simulink model "modelo"  (R2020a)
settings: Solver=FixedStepAuto  StartTime=0.0  StopTime=0.05  FixedStep=100e-9  RelTol=1e-3
values from neighbouring files (symbols this model uses):
  c1 = 220e-6    (= 0.00022)    [Untitled.m]
  c2 = 220e-6    (= 0.00022)    [Untitled.m]
  lb = 33e-6    (= 3.3e-05)    [Untitled.m]
  lr = 1.7e-6    (= 1.7e-06)    [Untitled.m]
  rb = 0.010    (= 0.01)    [Untitled.m]
  sc1 = 0.350    (= 0.35)    [Untitled.m]
  sc2 = 0.350    (= 0.35)    [Untitled.m]
  vb = 3.3    [Untitled.m]
  w = 2*pi*20e3    (= 125663.706144)    [Untitled.m]
libraries: powerlib x27
settings Model: Creator=nunin  LastModifiedBy=nunin

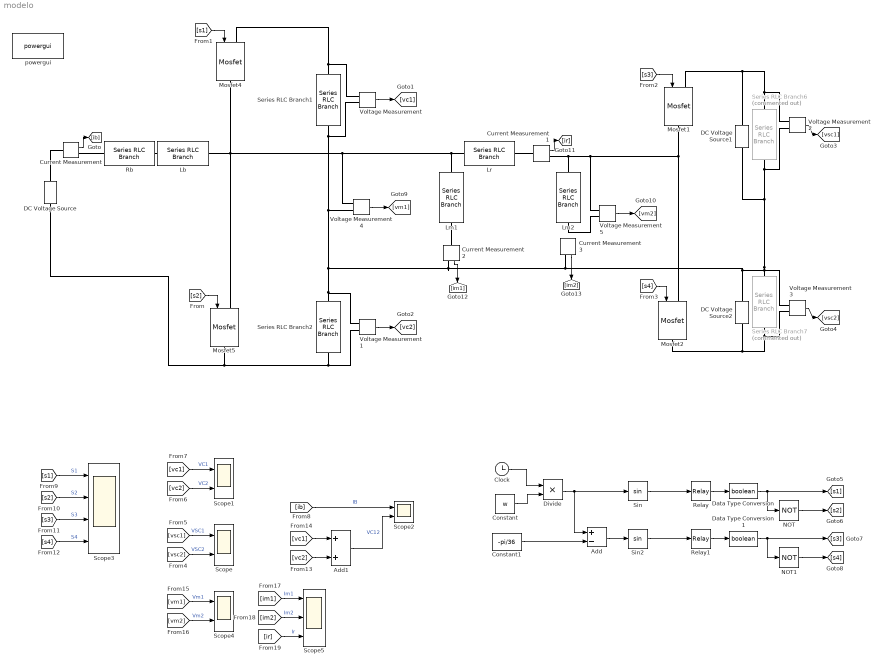
== system modelo ==
  Add : Sum  Inputs=+-
  Add1 : Sum
  Clock : Clock
  Constant : Constant  Value=w
  Constant1 : Constant  Value=-pi/36  VectorParams1D=off
  Current Measurement{,1..3} (4 alike) : powerlib/Measurements/Current Measurement  PhasorSimulation=off  OutputType=Complex  PSBequivalent=0
  DC Voltage Source : powerlib/Electrical Sources/DC Voltage Source  Amplitude=vb  Measurements=None
  DC Voltage Source1 : powerlib/Electrical Sources/DC Voltage Source  Amplitude=vb  Measurements=None
  DC Voltage Source2 : powerlib/Electrical Sources/DC Voltage Source  Amplitude=vb  Measurements=None
  Data Type Conversion : DataTypeConversion  OutDataTypeStr=boolean
  Data Type Conversion1 : DataTypeConversion  OutDataTypeStr=boolean
  Divide : Product  Inputs=**
  Lb : powerlib/Elements/Series RLC Branch  LConnTagsString=__new0  RConnTagsString=__new0  BranchType=L  Resistance=rb  Inductance=lb  SetiL0=off  InitialCurrent=0  Capacitance=1e-6  Setx0=off  InitialVoltage=0  Measurements=None
  Lm1 : powerlib/Elements/Series RLC Branch  LConnTagsString=__new0  RConnTagsString=__new0  BranchType=L  Resistance=rb  Inductance=1  SetiL0=off  InitialCurrent=0  Capacitance=1e-6  Setx0=off  InitialVoltage=0  Measurements=None
  Lm2 : powerlib/Elements/Series RLC Branch  LConnTagsString=__new0  RConnTagsString=__new0  BranchType=L  Resistance=rb  Inductance=1  SetiL0=off  InitialCurrent=0  Capacitance=1e-6  Setx0=off  InitialVoltage=0  Measurements=None
  Lr : powerlib/Elements/Series RLC Branch  LConnTagsString=__new0  RConnTagsString=__new0  BranchType=L  Resistance=rb  Inductance=lr  SetiL0=off  InitialCurrent=0  Capacitance=1e-6  Setx0=off  InitialVoltage=0  Measurements=None
  Mosfet{1..2,4..5} (4 alike) : powerlib/Power Electronics/Mosfet  Ron=1e-9  Lon=0  Rd=1e-9  Vfd=0  IC=0  Rs=1e10  Cs=inf  Measurements=off
  NOT : Logic  Operator=NOT  IconShape=distinctive  AllPortsSameDT=off  OutDataTypeStr=boolean
  NOT1 : Logic  Operator=NOT  IconShape=distinctive  AllPortsSameDT=off  OutDataTypeStr=boolean
  Rb : powerlib/Elements/Series RLC Branch  LConnTagsString=__new0  RConnTagsString=__new0  BranchType=R  Resistance=rb  Inductance=lb  SetiL0=off  InitialCurrent=0  Capacitance=1e-6  Setx0=off  InitialVoltage=0  Measurements=None
  Relay : Relay
  Relay1 : Relay
  Scope{,1..2,4} (4 alike) : Scope  NumInputPorts=2
  Scope3 : Scope  NumInputPorts=4
  Scope5 : Scope  NumInputPorts=3
  Series RLC Branch1 : powerlib/Elements/Series RLC Branch  LConnTagsString=__new0  RConnTagsString=__new0  BranchType=C  Resistance=rb  Inductance=lb  SetiL0=off  InitialCurrent=0  Capacitance=c1  Setx0=on  InitialVoltage=3.3  Measurements=None
  Series RLC Branch2 : powerlib/Elements/Series RLC Branch  LConnTagsString=__new0  RConnTagsString=__new0  BranchType=C  Resistance=rb  Inductance=lb  SetiL0=off  InitialCurrent=0  Capacitance=c2  Setx0=on  InitialVoltage=3.3  Measurements=None
  Series RLC Branch6 : powerlib/Elements/Series RLC Branch  Commented=on  LConnTagsString=__new0  RConnTagsString=__new0  BranchType=C  Resistance=rb  Inductance=lb  SetiL0=off  InitialCurrent=0  Capacitance=sc1  Setx0=on  InitialVoltage=3.3  Measurements=None
  Series RLC Branch7 : powerlib/Elements/Series RLC Branch  Commented=on  LConnTagsString=__new0  RConnTagsString=__new0  BranchType=C  Resistance=rb  Inductance=lb  SetiL0=off  InitialCurrent=0  Capacitance=sc2  Setx0=on  InitialVoltage=3.3  Measurements=None
  Sin : Trigonometry
  Sin2 : Trigonometry
  Voltage Measurement{,1..5} (6 alike) : powerlib/Measurements/Voltage Measurement  PhasorSimulation=off  OutputType=Complex  PSBequivalent=0
  powergui : powerlib/powergui  Priority=1  SimulationMode=Discrete  SampleTime=100e-9  frequency=60  Iterations=50  frequencyindice=0  Pbase=100e6  ErrMax=1e-4  UnitsV=kV  UnitsW=MW  buscounter=0  FunctionMessages=off  echomessages=off  EnableUseOfTLC=off  CurrentSourceSwitches=off  DisableSnubberDevices=off  DisableRonSwitches=off  DisableVfSwitches=off  DisplayEquations=off  AutomaticDiscreteSolvers=off  SolverType=Tustin/Backward Euler (TBE)  Interpol=off  ExternalGateDelay=off  methode=off  Ts=100  x0status=blocks  SPID=on  SwTol=0  HookPort=off  NonlinearTolerance=1e-4  nMaxIteration=100  ContinueOnMaxIteration=off  RestoreLinks=warning  ResistiveCurrentMeasurement=off  Frange=[0:2:500]  Ylog=off  Xlog=on  ShowGrid=off  save=off  variable=ZData  structure=0  ZoomFFT=off  StartTime=0.0  cycles=1  DisplayStyle=1  fundamental=60  FreqAxis=off  MaxFrequency=1000  frequencyindicesteady=1  RmsSteady=1  display=off
  wires:
  Current Measurement/1 -> [ib]
  Voltage Measurement/1 -> [vc1]
  Voltage Measurement1/1 -> [vc2]
  Voltage Measurement2/1 -> [vsc1]
  Voltage Measurement3/1 -> [vsc2]
  Clock/1 -> Divide/1
  Constant/1 -> Divide/2
  Divide/1 -> Add/1, Sin/1
  Constant1/1 -> Add/2
  Add/1 -> Sin2/1
  Sin/1 -> Relay/1
  Sin2/1 -> Relay1/1
  Relay/1 -> Data Type Conversion/1
  Data Type Conversion/1 -> NOT/1, [s1]
  NOT/1 -> [s2]
  NOT1/1 -> [s4]
  Data Type Conversion1/1 -> [s3], NOT1/1
  Relay1/1 -> Data Type Conversion1/1
  [s2] -> Mosfet5/1
  [s4] -> Mosfet2/1
  [s3] -> Mosfet1/1
  [s1] -> Mosfet4/1
  [vsc2] -> Scope/2  "VSC2"
  [vsc1] -> Scope/1  "VSC1"
  [vc2] -> Scope1/2  "VC2"
  [vc1] -> Scope1/1  "VC1"
  [ib] -> Scope2/1  "IB"
  [s1] -> Scope3/1  "S1"
  [s2] -> Scope3/2  "S2"
  [s4] -> Scope3/4  "S4"
  [s3] -> Scope3/3  "S3"
  [vc2] -> Add1/2
  [vc1] -> Add1/1
  Add1/1 -> Scope2/2  "VC12"
  Voltage Measurement4/1 -> [vm1]
  Voltage Measurement5/1 -> [vm2]
  [vm2] -> Scope4/2  "Vm2"
  [vm1] -> Scope4/1  "Vm1"
  Current Measurement1/1 -> [ir]
  Current Measurement2/1 -> [im1]
  Current Measurement3/1 -> [im2]
  [im1] -> Scope5/1  "Im1"
  [im2] -> Scope5/2  "Im2"
  [ir] -> Scope5/3  "Ir"
  connections:
  Rb/LConn1 -- Current Measurement/RConn1
  Current Measurement/LConn1 -- DC Voltage Source/RConn1
  Series RLC Branch1/LConn1 -- Mosfet4/LConn1 -- Voltage Measurement/LConn1
  Series RLC Branch2/RConn1 -- Mosfet5/RConn1 -- DC Voltage Source/LConn1 -- Voltage Measurement1/LConn2
  Lr/LConn1 -- Voltage Measurement4/LConn1 -- Mosfet5/LConn1 -- Mosfet4/RConn1 -- Lb/RConn1 -- Lm1/LConn1
  Voltage Measurement2/LConn1 -- Mosfet1/LConn1 -- DC Voltage Source1/RConn1 -- Series RLC Branch6/LConn1
  Voltage Measurement3/LConn2 -- Mosfet2/RConn1 -- DC Voltage Source2/LConn1 -- Series RLC Branch7/RConn1
  Series RLC Branch2/LConn1 -- Voltage Measurement1/LConn1 -- Current Measurement2/RConn1 -- Current Measurement3/RConn1 -- DC Voltage Source2/RConn1 -- Series RLC Branch7/LConn1 -- DC Voltage Source1/LConn1 -- Voltage Measurement2/LConn2 -- Series RLC Branch6/RConn1 -- Voltage Measurement3/LConn1 -- Voltage Measurement/LConn2 -- Series RLC Branch1/RConn1 -- Voltage Measurement4/LConn2
  Lb/LConn1 -- Rb/RConn1
  Voltage Measurement5/LConn1 -- Mosfet2/LConn1 -- Mosfet1/RConn1 -- Lm2/LConn1 -- Current Measurement1/RConn1
  Current Measurement1/LConn1 -- Lr/RConn1
  Current Measurement2/LConn1 -- Lm1/RConn1
  Lm2/RConn1 -- Voltage Measurement5/LConn2
